simulink model "dsp101"  (R2026b)
settings: Solver=FixedStepAuto  StopTime=10
libraries: androiduilib x9, androidcommunicationlib x6, androidsensorlib x3, simulink x2, androidaudiovideolib x2, simulink_extras x1
settings Model: Creator=rohan  LastModifiedBy=rohan
settings OptimizationCC: DefaultParameterBehavior=Inlined  DifferentSizesBufferReuse=on  EfficientTunableParamExpr=on  EnhancedBackFolding=on  MaxStackSize=64  OptimizationCustomize=off  OptimizeBlockOrder=speed  PassReuseOutputArgsAs=Individual arguments  RemoveInternalMemoryZeroInit=on  RemoveRootLevelIOMemoryZeroInit=on
settings DebuggingCC: ParameterTunabilityLossMsg=error
settings HardwareCC: ProdHWDeviceType=ARM Compatible->ARM Cortex-A (64-bit)  ProdLargestAtomicFloat=Double  ProdLargestAtomicInteger=LongLong  ProdLongLongMode=on  UseEmbeddedCoderFeatures=off  UseSimulinkCoderFeatures=off
settings SFSimCC: MATLABDynamicMemAlloc=off
settings RTWCC: Description=Embedded Coder  HardwareBoard=Android Device (64bit)  RTWVerbose=off  SystemTargetFile=ert.tlc  TLCOptions="-aInlineSetEventsForThisBaseRateFcn=TLC_FALSE -aSuppressMultiTaskScheduler=TLC_FALSE  -aRateBasedStepFcn=0"  TemplateMakefile=ert_default_tmf  Toolchain=Android SDK/NDK Tools
settings CodeAppCC: ForceParamTrailComments=on  IgnoreCustomStorageClasses=off  InsertBlockDesc=on  OperatorAnnotations=on  SFDataObjDesc=on  SimulinkDataObjDesc=on
settings ERTTargetCC: CombineSignalStateStructs=on  SupportNonInlinedSFcns=on

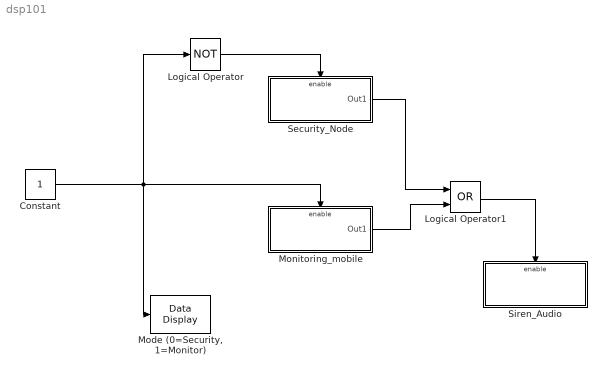
== system dsp101 ==
  Constant : Constant
  Logical Operator : Logic  Operator=NOT  Inputs=1  AllPortsSameDT=off  OutDataTypeStr=boolean
  Logical Operator1 : Logic  Operator=OR  AllPortsSameDT=off  OutDataTypeStr=boolean
  "Mode (0=Security, 1=Monitor)" : androiduilib/Data Display  DataDisplayId=dsp101/Mode_(0=Security,_1=Monitor)  Format=Float  Precision=6  SimulateUsing=Code generation  blockPlatform=Android
  Monitoring_mobile : Subsystem  TreatAsAtomicUnit=on
  Security_Node : Subsystem  TreatAsAtomicUnit=on
  Siren_Audio : Subsystem  TreatAsAtomicUnit=on
  wires:
  Constant/1 -> "Mode (0=Security, 1=Monitor)"/1, Logical Operator/1, Monitoring_mobile/Enable
  Logical Operator/1 -> Security_Node/Enable
  Security_Node/1(Out1) -> Logical Operator1/1
  Monitoring_mobile/1(Out1) -> Logical Operator1/2
  Logical Operator1/1 -> Siren_Audio/Enable

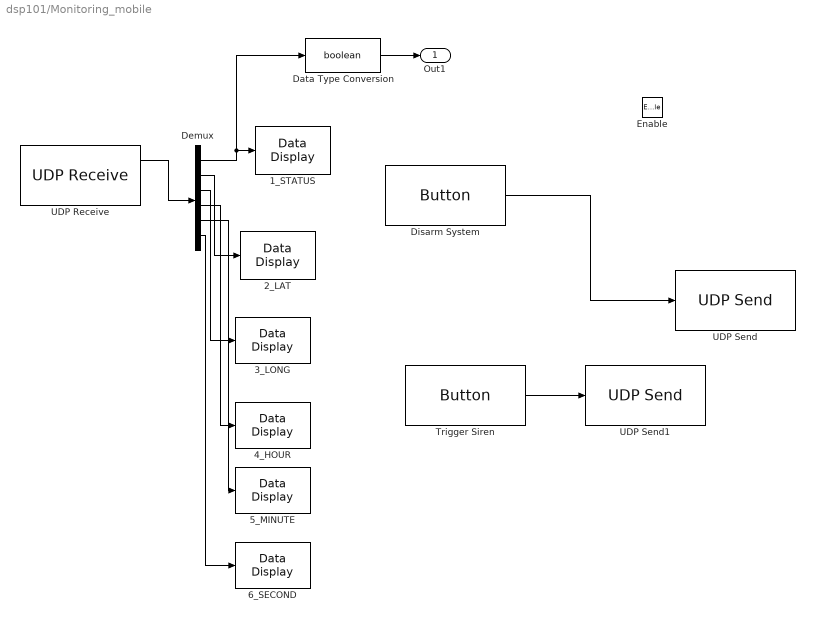
== system dsp101/Monitoring_mobile ==
  Enable : EnablePort
  1_STATUS : androiduilib/Data Display  DataDisplayId=dsp101/Monitoring_mobile/1_STATUS  Format=Float  Precision=6  SimulateUsing=Code generation  blockPlatform=Android
  2_LAT : androiduilib/Data Display  DataDisplayId=dsp101/Monitoring_mobile/2_LAT  Format=Float  Precision=6  SimulateUsing=Code generation  blockPlatform=Android
  3_LONG : androiduilib/Data Display  DataDisplayId=dsp101/Monitoring_mobile/3_LONG  Format=Float  Precision=6  SimulateUsing=Code generation  blockPlatform=Android
  4_HOUR : androiduilib/Data Display  DataDisplayId=dsp101/Monitoring_mobile/4_HOUR  Format=Float  Precision=6  SimulateUsing=Code generation  blockPlatform=Android
  5_MINUTE : androiduilib/Data Display  DataDisplayId=dsp101/Monitoring_mobile/5_MINUTE  Format=Float  Precision=6  SimulateUsing=Code generation  blockPlatform=Android
  6_SECOND : androiduilib/Data Display  DataDisplayId=dsp101/Monitoring_mobile/6_SECOND  Format=Float  Precision=6  SimulateUsing=Code generation  blockPlatform=Android
  Data Type Conversion : DataTypeConversion  OutDataTypeStr=boolean  SaturateOnIntegerOverflow=off  RndMeth=Floor
  Demux : Demux  Outputs=6
  Disarm System : androiduilib/Button  ButtonState=Not pressed  ButtonId=dsp101/Monitoring_mobile/Disarm_System  State=off  SampleTime=0.1  BlockPlatform=Android
  Trigger Siren : androiduilib/Button  ButtonState=Not pressed  ButtonId=dsp101/Monitoring_mobile/Trigger_Siren  State=off  SampleTime=0.1  BlockPlatform=Android
  UDP Receive : androidcommunicationlib/UDP Receive  localURL='0.0.0.0'  localPort=25000  remoteURL='0.0.0.0'  remotePort=-1  recvBufferSize=8192  signalDatatype=double  dims=6  isVarSize=off  showBlockingTime=off  blockingTime=0  sampletime=-1  blockPlatform=Android
  UDP Send : androidcommunicationlib/UDP Send  remoteURL='10.7.18.245'  remotePort=25001  localURL='0.0.0.0'  localPortSource=Automatically determine  localPort=-1  sampletime=-1  blockPlatform=Android  separateLengthPort=0
  UDP Send1 : androidcommunicationlib/UDP Send  remoteURL='10.7.18.245'  remotePort=25002  localURL='0.0.0.0'  localPortSource=Automatically determine  localPort=-1  sampletime=-1  blockPlatform=Android  separateLengthPort=0
  Out1 : Outport
  wires:
  UDP Receive/1 -> Demux/1
  Demux/1 -> Data Type Conversion/1, 1_STATUS/1
  Demux/3 -> 3_LONG/1
  Data Type Conversion/1 -> Out1/1
  Disarm System/1 -> UDP Send/1
  Trigger Siren/1 -> UDP Send1/1
  Demux/2 -> 2_LAT/1
  Demux/4 -> 4_HOUR/1
  Demux/5 -> 5_MINUTE/1
  Demux/6 -> 6_SECOND/1

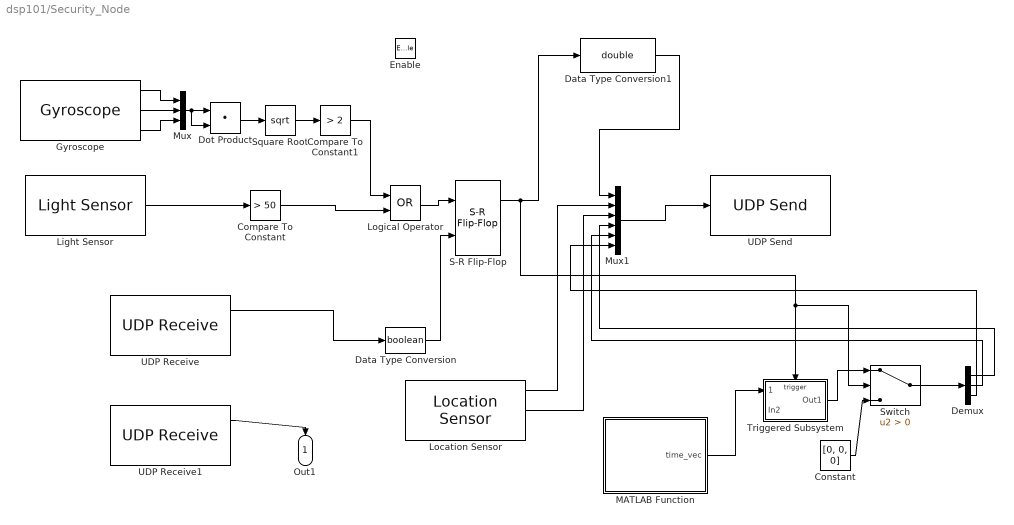
== system dsp101/Security_Node ==
  Enable : EnablePort
  Compare To Constant : simulink/Logic and Bit Operations/Compare To Constant  relop=>  const=50  OutDataTypeStr=boolean
  Compare To Constant1 : simulink/Logic and Bit Operations/Compare To Constant  relop=>  const=2  OutDataTypeStr=boolean
  Constant : Constant  Value=[0, 0, 0]
  Data Type Conversion : DataTypeConversion  OutDataTypeStr=boolean  SaturateOnIntegerOverflow=off  RndMeth=Floor
  Data Type Conversion1 : DataTypeConversion  OutDataTypeStr=double  SaturateOnIntegerOverflow=off  RndMeth=Floor
  Demux : Demux  Outputs=3
  Dot Product : DotProduct  OutDataTypeStr=Inherit: Inherit via internal rule
  Gyroscope : androidsensorlib/Gyroscope  OutputVector=off  SampleTime=0.1  BlockPlatform=Android
  Light Sensor : androidsensorlib/Light Sensor  SampleTime=0.1  BlockPlatform=Android
  Location Sensor : androidsensorlib/Location Sensor  OutputVector=off  SampleTime=0.1  BlockPlatform=Android
  Logical Operator : Logic  Operator=OR  AllPortsSameDT=off  OutDataTypeStr=boolean
  MATLAB Function : MATLAB Function  TreatAsAtomicUnit=on
  Mux : Mux  Inputs=3
  Mux1 : Mux  Inputs=6
  S-R Flip-Flop : simulink_extras/Flip Flops/S-R Flip-Flop  initial_condition=0
  Square Root : Sqrt
  Switch : Switch  Criteria=u2 > Threshold  SaturateOnIntegerOverflow=off  InputSameDT=off
  Triggered Subsystem : Subsystem  TreatAsAtomicUnit=on
  UDP Receive : androidcommunicationlib/UDP Receive  localURL='0.0.0.0'  localPort=25001  remoteURL='0.0.0.0'  remotePort=-1  recvBufferSize=8192  signalDatatype=double  dims=1  isVarSize=off  showBlockingTime=off  blockingTime=0  sampletime=-1  blockPlatform=Android
  UDP Receive1 : androidcommunicationlib/UDP Receive  localURL='0.0.0.0'  localPort=25002  remoteURL='0.0.0.0'  remotePort=-1  recvBufferSize=8192  signalDatatype=double  dims=1  isVarSize=off  showBlockingTime=off  blockingTime=0  sampletime=-1  blockPlatform=Android
  UDP Send : androidcommunicationlib/UDP Send  remoteURL='10.7.31.222'  remotePort=25000  localURL='0.0.0.0'  localPortSource=Automatically determine  localPort=-1  sampletime=-1  blockPlatform=Android  separateLengthPort=0
  Out1 : Outport
  wires:
  Light Sensor/1 -> Compare To Constant/1
  Gyroscope/1 -> Mux/1
  Gyroscope/2 -> Mux/2
  Gyroscope/3 -> Mux/3
  Mux/1 -> Dot Product/2, Dot Product/1
  Dot Product/1 -> Square Root/1
  Square Root/1 -> Compare To Constant1/1
  Compare To Constant1/1 -> Logical Operator/1
  Logical Operator/1 -> S-R Flip-Flop/1
  S-R Flip-Flop/1 -> Switch/2, Triggered Subsystem/Trigger, Data Type Conversion1/1
  Location Sensor/1 -> Mux1/2
  Location Sensor/2 -> Mux1/3
  Mux1/1 -> UDP Send/1
  Data Type Conversion/1 -> S-R Flip-Flop/2
  Data Type Conversion1/1 -> Mux1/1
  Triggered Subsystem/1(Out1) -> Switch/1
  Constant/1 -> Switch/3
  UDP Receive/1 -> Data Type Conversion/1
  UDP Receive1/1 -> Out1/1
  MATLAB Function/1(time_vec) -> Triggered Subsystem/1(hhmmss)
  Switch/1 -> Demux/1
  Demux/1 -> Mux1/4
  Demux/2 -> Mux1/5
  Demux/3 -> Mux1/6
  Compare To Constant/1 -> Logical Operator/2

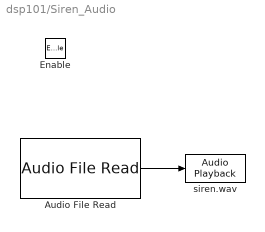
== system dsp101/Siren_Audio ==
  Enable : EnablePort
  Audio File Read : androidaudiovideolib/Audio File Read  FileName=C:\Matlab_projects\siren.wav  FrameSize=4410
  siren.wav : androidaudiovideolib/Audio Playback  SampleFreq=44100  AudioSamplingFreq=44100  SampleTime=0.1  DeviceStr=0  QueueDuration=0  BlockPlatform=Android
  wires:
  Audio File Read/1 -> siren.wav/1

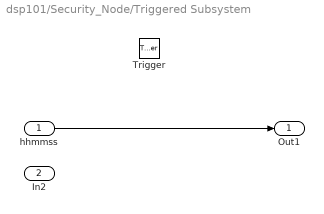
== system dsp101/Security_Node/Triggered Subsystem ==
  hhmmss : Inport
  In2 : Inport  Port=2
  Trigger : TriggerPort  VariantControl=(inherit)
  Out1 : Outport
  wires:
  hhmmss/1 -> Out1/1

== matlab function dsp101/Security_Node/MATLAB Function ==
  data: time_vec output
function time_vec = get_device_time()
%#codegen
coder.cinclude('<time.h>');

unix_sec = double(0);
if coder.target('Rtw')
    unix_sec = coder.ceval('time', coder.opaque('void*', 'NULL'));
end

local_sec = unix_sec + 19800;
sec_today = mod(local_sec, 86400);
h = floor(sec_today / 3600);
m = floor(mod(sec_today, 3600) / 60);
s = floor(mod(sec_today, 60));

% Output as a 1x3 array: [Hours, Minutes, Seconds]
time_vec = [h, m, s];
